simulink model "tackingSim"  (R2022b)
settings: Solver=FixedStepAuto  StartTime=0.0  StopTime=20  FixedStep=0.01  RelTol=1e-3
settings Model: Creator=ruben  LastModifiedBy=ruben

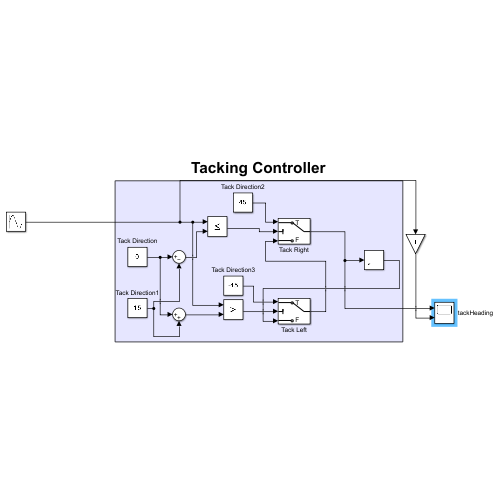
[thumbnail: Simulink's stored preview of the top-level diagram]
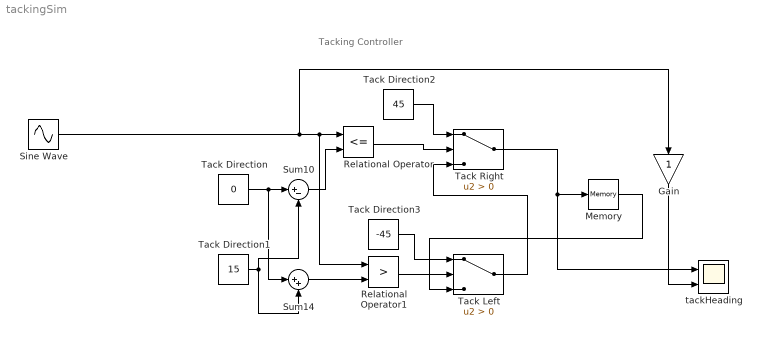
== system tackingSim ==
  note: Tacking Controller
  Gain : Gain
  Memory : Memory
  Relational Operator : RelationalOperator  Operator=<=  OutDataTypeStr=boolean  RndMeth=Simplest  InputSameDT=off
  Relational Operator1 : RelationalOperator  Operator=>  OutDataTypeStr=boolean  RndMeth=Simplest  InputSameDT=off
  Sine Wave : Sin  Amplitude=17.5  SampleTime=0
  Sum10 : Sum  Inputs=|+-
  Sum14 : Sum  Inputs=|++
  Tack Direction : Constant  Value=0
  Tack Direction1 : Constant  Value=15
  Tack Direction2 : Constant  Value=45
  Tack Direction3 : Constant  Value=-45
  Tack Left : Switch  Criteria=u2 > Threshold  SaturateOnIntegerOverflow=off  InputSameDT=off
  Tack Right : Switch  Criteria=u2 > Threshold  SaturateOnIntegerOverflow=off  InputSameDT=off
  tackHeading : Scope  NumInputPorts=2
  wires:
  Sum14/1 -> Relational Operator1/2
  Tack Right/1 -> Memory/1, tackHeading/1
  Tack Direction/1 -> Sum14/1, Sum10/1
  Memory/1 -> Tack Left/3
  Sum10/1 -> Relational Operator/2
  Relational Operator/1 -> Tack Right/2
  Relational Operator1/1 -> Tack Left/2
  Tack Left/1 -> Tack Right/3
  Tack Direction1/1 -> Sum10/2, Sum14/2
  Sine Wave/1 -> Gain/1, Relational Operator1/1, Relational Operator/1
  Tack Direction3/1 -> Tack Left/1
  Tack Direction2/1 -> Tack Right/1
  Gain/1 -> tackHeading/2
